simulink model "Md58TrgtPos"  (R2018b)
settings: Solver=FixedStepDiscrete  StartTime=0.0  StopTime=10.0  RelTol=1e-3
undefined symbols (not defined in the file or in its folder): arg, Rte_EEP_Md58PassStBkReclnTrgtPos_Set, Rte_EEP_Md58PassStFldTrgtPos_Set, Rte_EEP_Md58PassStFwdBkwdTrgtPos_Set, Rte_EEP_Md58SecRwRtStBkReclnTrgtPos_Set, Rte_EEP_Md58SecRwRtStCushFrntTrgtPos_Set, Rte_EEP_Md58SecRwRtStFwdBkwdTrgtPos_Set, Rte_EEP_Md58SecRwRtStLgrstInwdOtwdTrgtPos_Set, Rte_EEP_Md58SecRwRtStLgrstUpwdDnwdTrgtPos_Set, Rte_EEP_Md58ThdRwLtStBkReclnTrgtPos_Set, Rte_EEP_Md58ThdRwLtStFwdBkwdTrgtPos_Set, Rte_EEP_Md58ThdRwRtStBkReclnTrgtPos_Set, Rte_EEP_Md58ThdRwRtStFwdBkwdTrgtPos_Set
settings Model: ModifiedHistory=2024.10.14 V3.0.0 新增Md58  Creator=sn2xws  LastModifiedBy=sn2xws
settings DataIOCC: SaveFormat=StructureWithTime
settings OptimizationCC: DefaultParameterBehavior=Inlined  EnhancedBackFolding=on  PassReuseOutputArgsAs=Individual arguments  ZeroExternalMemoryAtStartup=off  ZeroInternalMemoryAtStartup=off  OptimizeBlockOrder=speed  DifferentSizesBufferReuse=on  OptimizationCustomize=off
settings DebuggingCC: ParameterTunabilityLossMsg=error
settings SFSimCC: MATLABDynamicMemAlloc=off
settings RTWCC: SystemTargetFile=autosar.tlc  GenCodeOnly=on  TemplateMakefile=ert_default_tmf  Description=AUTOSAR  GenerateReport=on  IncludeHyperlinkInReport=on  LaunchReport=on  GenerateTraceInfo=on  GenerateTraceReport=on  GenerateTraceReportSl=on  GenerateTraceReportSf=on  GenerateTraceReportEml=on
settings CodeAppCC: ForceParamTrailComments=on  IgnoreCustomStorageClasses=off  OperatorAnnotations=on  SimulinkDataObjDesc=on  SFDataObjDesc=on  InsertBlockDesc=on
settings STFCustomTargetCC: TargetLangStandard=C99 (ISO)  MultiwordLength=256  ParMdlRefBuildCompliant=on  CompOptLevelCompliant=on  IncludeMdlTerminateFcn=off  CombineOutputUpdateFcns=on  SuppressErrorStatus=on  ERTCustomFileBanners=on  SupportNonFinite=off  SupportComplex=off  SupportContinuousTime=off  SupportNonInlinedSFcns=off  RemoveResetFunc=on  MATLABClassNameForMDSCustomization=Simulink.SoftwareTarget.ERTCustomization  AutosarCompliant=on  UseToolchainInfoCompliant=on  LookupTableObjectStructAxisOrder=2,1,3,4,...  LUTObjectStructOrderEvenSpacing=Size,Table,Breakpoints  SystemTargetFile=autosar.tlc
settings ERTTargetCC: TargetLangStandard=C99 (ISO)  ConcurrentExecutionCompliant=off  IncludeMdlTerminateFcn=off  SuppressErrorStatus=on  SupportNonFinite=off  SupportComplex=off  ModelStepFunctionPrototypeControlCompliant=off  CPPClassGenCompliant=off  AutosarCompliant=on  LookupTableObjectStructAxisOrder=2,1,3,4,...  LUTObjectStructOrderEvenSpacing=Size,Table,Breakpoints  InlinedParameterPlacement=NonHierarchical  ERTCustomFileTemplate=example_file_process.tlc  ERTFilePackagingFormat=Compact

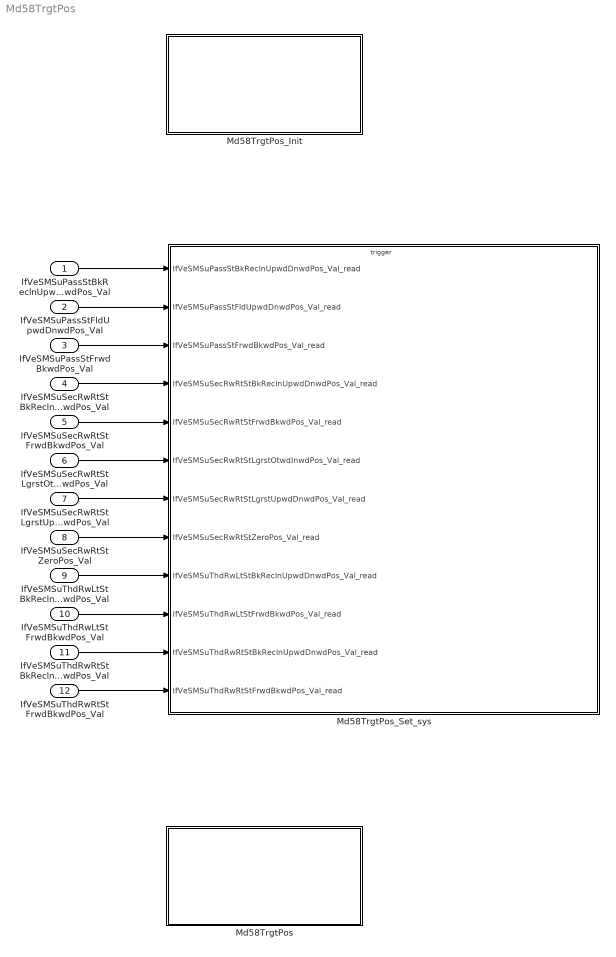
== system Md58TrgtPos ==
  IfVeSMSuPassStBkReclnUpwdDnwdPos_Val : Inport  OutDataTypeStr=uint16  PortDimensions=1
  IfVeSMSuPassStFldUpwdDnwdPos_Val : Inport  Port=2  OutDataTypeStr=uint16  PortDimensions=1
  IfVeSMSuPassStFrwdBkwdPos_Val : Inport  Port=3  OutDataTypeStr=uint16  PortDimensions=1
  IfVeSMSuSecRwRtStBkReclnUpwdDnwdPos_Val : Inport  Port=4  OutDataTypeStr=uint16  PortDimensions=1
  IfVeSMSuSecRwRtStFrwdBkwdPos_Val : Inport  Port=5  OutDataTypeStr=uint16  PortDimensions=1
  IfVeSMSuSecRwRtStLgrstOtwdInwdPos_Val : Inport  Port=6  OutDataTypeStr=uint16  PortDimensions=1
  IfVeSMSuSecRwRtStLgrstUpwdDnwdPos_Val : Inport  Port=7  OutDataTypeStr=uint16  PortDimensions=1
  IfVeSMSuSecRwRtStZeroPos_Val : Inport  Port=8  OutDataTypeStr=uint16  PortDimensions=1
  IfVeSMSuThdRwLtStBkReclnUpwdDnwdPos_Val : Inport  Port=9  OutDataTypeStr=uint16  PortDimensions=1
  IfVeSMSuThdRwLtStFrwdBkwdPos_Val : Inport  Port=10  OutDataTypeStr=uint16  PortDimensions=1
  IfVeSMSuThdRwRtStBkReclnUpwdDnwdPos_Val : Inport  Port=11  OutDataTypeStr=uint16  PortDimensions=1
  IfVeSMSuThdRwRtStFrwdBkwdPos_Val : Inport  Port=12  OutDataTypeStr=uint16  PortDimensions=1
  Md58TrgtPos : Subsystem
  Md58TrgtPos_Init : Subsystem
  Md58TrgtPos_Set_sys : Subsystem
  wires:
  IfVeSMSuPassStBkReclnUpwdDnwdPos_Val/1 -> Md58TrgtPos_Set_sys/1(IfVeSMSuPassStBkReclnUpwdDnwdPos_Val_read)
  IfVeSMSuPassStFldUpwdDnwdPos_Val/1 -> Md58TrgtPos_Set_sys/2(IfVeSMSuPassStFldUpwdDnwdPos_Val_read)
  IfVeSMSuPassStFrwdBkwdPos_Val/1 -> Md58TrgtPos_Set_sys/3(IfVeSMSuPassStFrwdBkwdPos_Val_read)
  IfVeSMSuSecRwRtStBkReclnUpwdDnwdPos_Val/1 -> Md58TrgtPos_Set_sys/4(IfVeSMSuSecRwRtStBkReclnUpwdDnwdPos_Val_read)
  IfVeSMSuSecRwRtStFrwdBkwdPos_Val/1 -> Md58TrgtPos_Set_sys/5(IfVeSMSuSecRwRtStFrwdBkwdPos_Val_read)
  IfVeSMSuSecRwRtStLgrstOtwdInwdPos_Val/1 -> Md58TrgtPos_Set_sys/6(IfVeSMSuSecRwRtStLgrstOtwdInwdPos_Val_read)
  IfVeSMSuSecRwRtStLgrstUpwdDnwdPos_Val/1 -> Md58TrgtPos_Set_sys/7(IfVeSMSuSecRwRtStLgrstUpwdDnwdPos_Val_read)
  IfVeSMSuSecRwRtStZeroPos_Val/1 -> Md58TrgtPos_Set_sys/8(IfVeSMSuSecRwRtStZeroPos_Val_read)
  IfVeSMSuThdRwLtStBkReclnUpwdDnwdPos_Val/1 -> Md58TrgtPos_Set_sys/9(IfVeSMSuThdRwLtStBkReclnUpwdDnwdPos_Val_read)
  IfVeSMSuThdRwLtStFrwdBkwdPos_Val/1 -> Md58TrgtPos_Set_sys/10(IfVeSMSuThdRwLtStFrwdBkwdPos_Val_read)
  IfVeSMSuThdRwRtStBkReclnUpwdDnwdPos_Val/1 -> Md58TrgtPos_Set_sys/11(IfVeSMSuThdRwRtStBkReclnUpwdDnwdPos_Val_read)
  IfVeSMSuThdRwRtStFrwdBkwdPos_Val/1 -> Md58TrgtPos_Set_sys/12(IfVeSMSuThdRwRtStFrwdBkwdPos_Val_read)

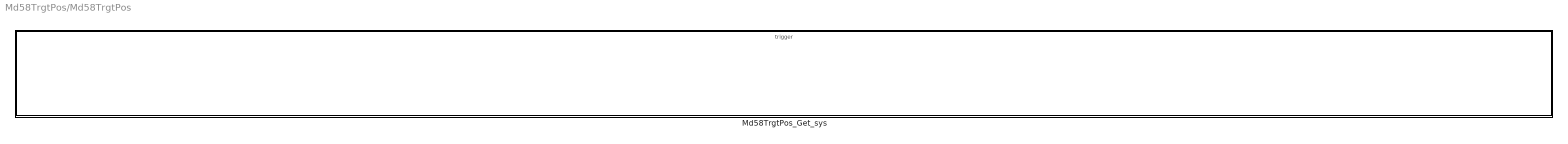
== system Md58TrgtPos/Md58TrgtPos ==
  Md58TrgtPos_Get_sys : Subsystem

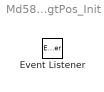
== system Md58TrgtPos/Md58TrgtPos_Init ==
  Event Listener : EventListener  EventName=reset

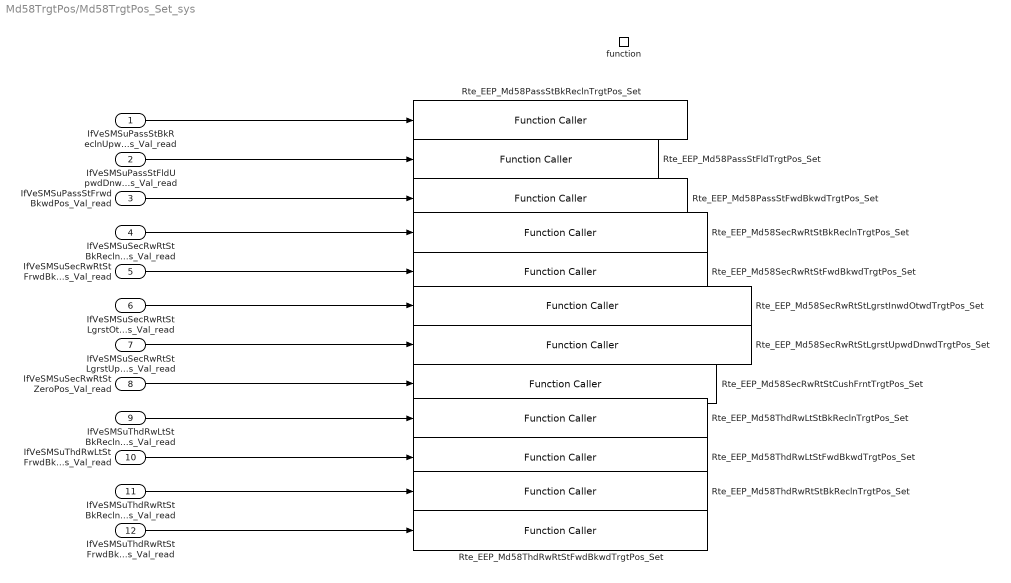
== system Md58TrgtPos/Md58TrgtPos_Set_sys ==
  IfVeSMSuPassStBkReclnUpwdDnwdPos_Val_read : Inport
  IfVeSMSuPassStFldUpwdDnwdPos_Val_read : Inport  Port=2
  IfVeSMSuPassStFrwdBkwdPos_Val_read : Inport  Port=3
  IfVeSMSuSecRwRtStBkReclnUpwdDnwdPos_Val_read : Inport  Port=4
  IfVeSMSuSecRwRtStFrwdBkwdPos_Val_read : Inport  Port=5
  IfVeSMSuSecRwRtStLgrstOtwdInwdPos_Val_read : Inport  Port=6
  IfVeSMSuSecRwRtStLgrstUpwdDnwdPos_Val_read : Inport  Port=7
  IfVeSMSuSecRwRtStZeroPos_Val_read : Inport  Port=8
  IfVeSMSuThdRwLtStBkReclnUpwdDnwdPos_Val_read : Inport  Port=9
  IfVeSMSuThdRwLtStFrwdBkwdPos_Val_read : Inport  Port=10
  IfVeSMSuThdRwRtStBkReclnUpwdDnwdPos_Val_read : Inport  Port=11
  IfVeSMSuThdRwRtStFrwdBkwdPos_Val_read : Inport  Port=12
  function : TriggerPort  TriggerType=function-call  IsSimulinkFunction=on  FunctionName=Md58TrgtPos_Set  VariantControl=(inherit)
  Rte_EEP_Md58PassStBkReclnTrgtPos_Set : FunctionCaller  FunctionPrototype=Rte_EEP_Md58PassStBkReclnTrgtPos_Set(arg)  InputArgumentSpecifications=P_EEP_Uint16
  Rte_EEP_Md58PassStFldTrgtPos_Set : FunctionCaller  FunctionPrototype=Rte_EEP_Md58PassStFldTrgtPos_Set(arg)  InputArgumentSpecifications=P_EEP_Uint16
  Rte_EEP_Md58PassStFwdBkwdTrgtPos_Set : FunctionCaller  FunctionPrototype=Rte_EEP_Md58PassStFwdBkwdTrgtPos_Set(arg)  InputArgumentSpecifications=P_EEP_Uint16
  Rte_EEP_Md58SecRwRtStBkReclnTrgtPos_Set : FunctionCaller  FunctionPrototype=Rte_EEP_Md58SecRwRtStBkReclnTrgtPos_Set(arg)  InputArgumentSpecifications=P_EEP_Uint16
  Rte_EEP_Md58SecRwRtStCushFrntTrgtPos_Set : FunctionCaller  FunctionPrototype=Rte_EEP_Md58SecRwRtStCushFrntTrgtPos_Set(arg)  InputArgumentSpecifications=P_EEP_Uint16
  Rte_EEP_Md58SecRwRtStFwdBkwdTrgtPos_Set : FunctionCaller  FunctionPrototype=Rte_EEP_Md58SecRwRtStFwdBkwdTrgtPos_Set(arg)  InputArgumentSpecifications=P_EEP_Uint16
  Rte_EEP_Md58SecRwRtStLgrstInwdOtwdTrgtPos_Set : FunctionCaller  FunctionPrototype=Rte_EEP_Md58SecRwRtStLgrstInwdOtwdTrgtPos_Set(arg)  InputArgumentSpecifications=P_EEP_Uint16
  Rte_EEP_Md58SecRwRtStLgrstUpwdDnwdTrgtPos_Set : FunctionCaller  FunctionPrototype=Rte_EEP_Md58SecRwRtStLgrstUpwdDnwdTrgtPos_Set(arg)  InputArgumentSpecifications=P_EEP_Uint16
  Rte_EEP_Md58ThdRwLtStBkReclnTrgtPos_Set : FunctionCaller  FunctionPrototype=Rte_EEP_Md58ThdRwLtStBkReclnTrgtPos_Set(arg)  InputArgumentSpecifications=P_EEP_Uint16
  Rte_EEP_Md58ThdRwLtStFwdBkwdTrgtPos_Set : FunctionCaller  FunctionPrototype=Rte_EEP_Md58ThdRwLtStFwdBkwdTrgtPos_Set(arg)  InputArgumentSpecifications=P_EEP_Uint16
  Rte_EEP_Md58ThdRwRtStBkReclnTrgtPos_Set : FunctionCaller  FunctionPrototype=Rte_EEP_Md58ThdRwRtStBkReclnTrgtPos_Set(arg)  InputArgumentSpecifications=P_EEP_Uint16
  Rte_EEP_Md58ThdRwRtStFwdBkwdTrgtPos_Set : FunctionCaller  FunctionPrototype=Rte_EEP_Md58ThdRwRtStFwdBkwdTrgtPos_Set(arg)  InputArgumentSpecifications=P_EEP_Uint16
  wires:
  IfVeSMSuPassStBkReclnUpwdDnwdPos_Val_read/1 -> Rte_EEP_Md58PassStBkReclnTrgtPos_Set/1
  IfVeSMSuPassStFrwdBkwdPos_Val_read/1 -> Rte_EEP_Md58PassStFwdBkwdTrgtPos_Set/1
  IfVeSMSuPassStFldUpwdDnwdPos_Val_read/1 -> Rte_EEP_Md58PassStFldTrgtPos_Set/1
  IfVeSMSuSecRwRtStBkReclnUpwdDnwdPos_Val_read/1 -> Rte_EEP_Md58SecRwRtStBkReclnTrgtPos_Set/1
  IfVeSMSuSecRwRtStZeroPos_Val_read/1 -> Rte_EEP_Md58SecRwRtStCushFrntTrgtPos_Set/1
  IfVeSMSuSecRwRtStFrwdBkwdPos_Val_read/1 -> Rte_EEP_Md58SecRwRtStFwdBkwdTrgtPos_Set/1
  IfVeSMSuSecRwRtStLgrstOtwdInwdPos_Val_read/1 -> Rte_EEP_Md58SecRwRtStLgrstInwdOtwdTrgtPos_Set/1
  IfVeSMSuSecRwRtStLgrstUpwdDnwdPos_Val_read/1 -> Rte_EEP_Md58SecRwRtStLgrstUpwdDnwdTrgtPos_Set/1
  IfVeSMSuThdRwLtStBkReclnUpwdDnwdPos_Val_read/1 -> Rte_EEP_Md58ThdRwLtStBkReclnTrgtPos_Set/1
  IfVeSMSuThdRwLtStFrwdBkwdPos_Val_read/1 -> Rte_EEP_Md58ThdRwLtStFwdBkwdTrgtPos_Set/1
  IfVeSMSuThdRwRtStBkReclnUpwdDnwdPos_Val_read/1 -> Rte_EEP_Md58ThdRwRtStBkReclnTrgtPos_Set/1
  IfVeSMSuThdRwRtStFrwdBkwdPos_Val_read/1 -> Rte_EEP_Md58ThdRwRtStFwdBkwdTrgtPos_Set/1

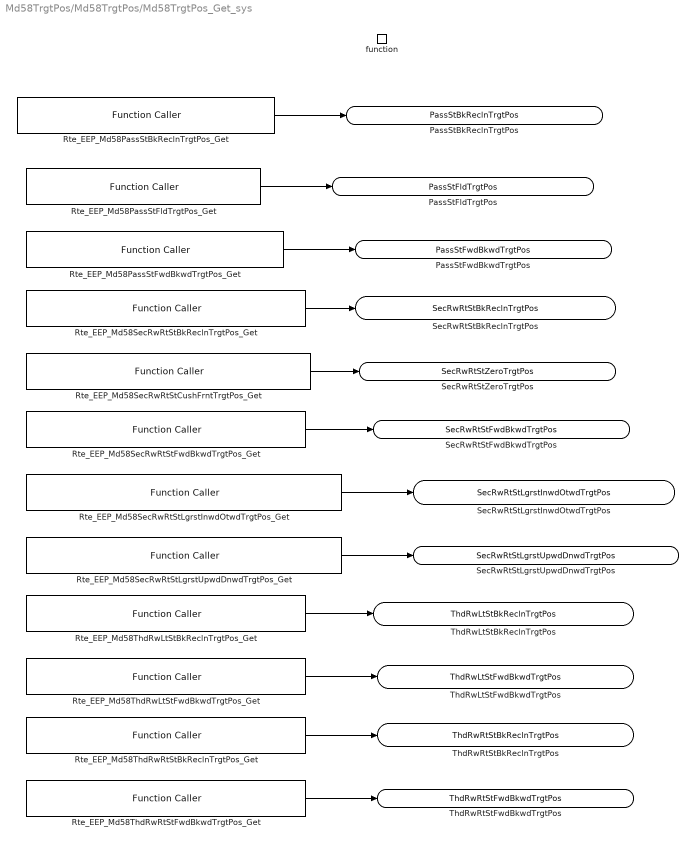
== system Md58TrgtPos/Md58TrgtPos/Md58TrgtPos_Get_sys ==
  function : TriggerPort  TriggerType=function-call  IsSimulinkFunction=on  FunctionName=Md58TrgtPos_Get  VariantControl=(inherit)
  Rte_EEP_Md58PassStBkReclnTrgtPos_Get : FunctionCaller  FunctionPrototype=arg = Rte_EEP_Md58PassStBkReclnTrgtPos_Get()  OutputArgumentSpecifications=P_EEP_Uint16
  Rte_EEP_Md58PassStFldTrgtPos_Get : FunctionCaller  FunctionPrototype=arg = Rte_EEP_Md58PassStFldTrgtPos_Get()  OutputArgumentSpecifications=P_EEP_Uint16
  Rte_EEP_Md58PassStFwdBkwdTrgtPos_Get : FunctionCaller  FunctionPrototype=arg = Rte_EEP_Md58PassStFwdBkwdTrgtPos_Get()  OutputArgumentSpecifications=P_EEP_Uint16
  Rte_EEP_Md58SecRwRtStBkReclnTrgtPos_Get : FunctionCaller  FunctionPrototype=arg = Rte_EEP_Md58SecRwRtStBkReclnTrgtPos_Get()  OutputArgumentSpecifications=P_EEP_Uint16
  Rte_EEP_Md58SecRwRtStCushFrntTrgtPos_Get : FunctionCaller  FunctionPrototype=arg = Rte_EEP_Md58SecRwRtStCushFrntTrgtPos_Get()  OutputArgumentSpecifications=P_EEP_Uint16
  Rte_EEP_Md58SecRwRtStFwdBkwdTrgtPos_Get : FunctionCaller  FunctionPrototype=arg = Rte_EEP_Md58SecRwRtStFwdBkwdTrgtPos_Get()  OutputArgumentSpecifications=P_EEP_Uint16
  Rte_EEP_Md58SecRwRtStLgrstInwdOtwdTrgtPos_Get : FunctionCaller  FunctionPrototype=arg = Rte_EEP_Md58SecRwRtStLgrstInwdOtwdTrgtPos_Get()  OutputArgumentSpecifications=P_EEP_Uint16
  Rte_EEP_Md58SecRwRtStLgrstUpwdDnwdTrgtPos_Get : FunctionCaller  FunctionPrototype=arg = Rte_EEP_Md58SecRwRtStLgrstUpwdDnwdTrgtPos_Get()  OutputArgumentSpecifications=P_EEP_Uint16
  Rte_EEP_Md58ThdRwLtStBkReclnTrgtPos_Get : FunctionCaller  FunctionPrototype=arg = Rte_EEP_Md58ThdRwLtStBkReclnTrgtPos_Get()  OutputArgumentSpecifications=P_EEP_Uint16
  Rte_EEP_Md58ThdRwLtStFwdBkwdTrgtPos_Get : FunctionCaller  FunctionPrototype=arg = Rte_EEP_Md58ThdRwLtStFwdBkwdTrgtPos_Get()  OutputArgumentSpecifications=P_EEP_Uint16
  Rte_EEP_Md58ThdRwRtStBkReclnTrgtPos_Get : FunctionCaller  FunctionPrototype=arg = Rte_EEP_Md58ThdRwRtStBkReclnTrgtPos_Get()  OutputArgumentSpecifications=P_EEP_Uint16
  Rte_EEP_Md58ThdRwRtStFwdBkwdTrgtPos_Get : FunctionCaller  FunctionPrototype=arg = Rte_EEP_Md58ThdRwRtStFwdBkwdTrgtPos_Get()  OutputArgumentSpecifications=P_EEP_Uint16
  SecRwRtStBkReclnTrgtPos : ArgOut  OutDataTypeStr=uint16  ArgumentName=SecRwRtStBkReclnTrgtPos
  SecRwRtStZeroTrgtPos : ArgOut  Port=2  OutDataTypeStr=uint16  ArgumentName=SecRwRtStZeroTrgtPos
  SecRwRtStLgrstUpwdDnwdTrgtPos : ArgOut  Port=3  OutDataTypeStr=uint16  ArgumentName=SecRwRtStLgrstUpwdDnwdTrgtPos
  SecRwRtStLgrstInwdOtwdTrgtPos : ArgOut  Port=4  OutDataTypeStr=uint16  ArgumentName=SecRwRtStLgrstInwdOtwdTrgtPos
  ThdRwLtStBkReclnTrgtPos : ArgOut  Port=5  OutDataTypeStr=uint16  ArgumentName=ThdRwLtStBkReclnTrgtPos
  ThdRwLtStFwdBkwdTrgtPos : ArgOut  Port=6  OutDataTypeStr=uint16  ArgumentName=ThdRwLtStFwdBkwdTrgtPos
  ThdRwRtStBkReclnTrgtPos : ArgOut  Port=7  OutDataTypeStr=uint16  ArgumentName=ThdRwRtStBkReclnTrgtPos
  ThdRwRtStFwdBkwdTrgtPos : ArgOut  Port=8  OutDataTypeStr=uint16  ArgumentName=ThdRwRtStFwdBkwdTrgtPos
  PassStBkReclnTrgtPos : ArgOut  Port=9  OutDataTypeStr=uint16  ArgumentName=PassStBkReclnTrgtPos
  PassStFwdBkwdTrgtPos : ArgOut  Port=10  OutDataTypeStr=uint16  ArgumentName=PassStFwdBkwdTrgtPos
  SecRwRtStFwdBkwdTrgtPos : ArgOut  Port=11  OutDataTypeStr=uint16  ArgumentName=SecRwRtStFwdBkwdTrgtPos
  PassStFldTrgtPos : ArgOut  Port=12  OutDataTypeStr=uint16  ArgumentName=PassStFldTrgtPos
  wires:
  Rte_EEP_Md58SecRwRtStCushFrntTrgtPos_Get/1 -> SecRwRtStZeroTrgtPos/1
  Rte_EEP_Md58SecRwRtStLgrstUpwdDnwdTrgtPos_Get/1 -> SecRwRtStLgrstUpwdDnwdTrgtPos/1
  Rte_EEP_Md58SecRwRtStLgrstInwdOtwdTrgtPos_Get/1 -> SecRwRtStLgrstInwdOtwdTrgtPos/1
  Rte_EEP_Md58ThdRwLtStBkReclnTrgtPos_Get/1 -> ThdRwLtStBkReclnTrgtPos/1
  Rte_EEP_Md58ThdRwLtStFwdBkwdTrgtPos_Get/1 -> ThdRwLtStFwdBkwdTrgtPos/1
  Rte_EEP_Md58ThdRwRtStBkReclnTrgtPos_Get/1 -> ThdRwRtStBkReclnTrgtPos/1
  Rte_EEP_Md58ThdRwRtStFwdBkwdTrgtPos_Get/1 -> ThdRwRtStFwdBkwdTrgtPos/1
  Rte_EEP_Md58PassStBkReclnTrgtPos_Get/1 -> PassStBkReclnTrgtPos/1
  Rte_EEP_Md58PassStFwdBkwdTrgtPos_Get/1 -> PassStFwdBkwdTrgtPos/1
  Rte_EEP_Md58SecRwRtStFwdBkwdTrgtPos_Get/1 -> SecRwRtStFwdBkwdTrgtPos/1
  Rte_EEP_Md58PassStFldTrgtPos_Get/1 -> PassStFldTrgtPos/1
  Rte_EEP_Md58SecRwRtStBkReclnTrgtPos_Get/1 -> SecRwRtStBkReclnTrgtPos/1
